simulink model "amuntitled"  (R2016a)
settings: Solver=FixedStepDiscrete  SolverMode=SingleTasking  StartTime=0.0  StopTime=4e-6  RelTol=1e-3
InitFcn:
  | %% DSPBuilder Start
  | alt_dspbuilder_update_model(bdroot)
  | %% DSPBuilder End
StartFcn:
  | %% DSPBuilder Start
  | alt_dspbuilder_hdlimport_prepare_for_simulation(bdroot)
  | %% DSPBuilder End
libraries: allblocks_alteradspbuilder2 x13
settings Model: Creator=ASUS  LastModifiedBy=ASUS

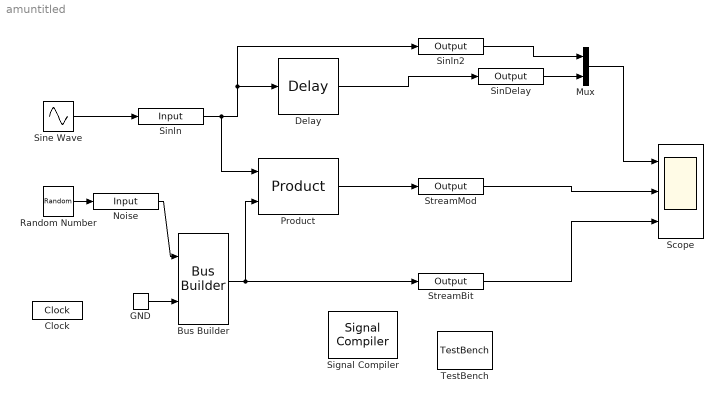
== system amuntitled ==
  Bus Builder : allblocks_alteradspbuilder2/Bus Builder  BusType=Signed Integer  bwl=2  bwr=1  pipeline_display=0
  Clock : allblocks_alteradspbuilder2/Clock  ClockPeriod=20  ClockPeriodUnit=ns  SampleTime=2.5e-008  ResetLatency=0  ResetRegisterCascadeDepth=0  SimulationStartCycle=5  PhaseOffset=0  Reset=aclr  ResetType=Active High  Export=off
  Delay : allblocks_alteradspbuilder2/Delay  pipeline=01  pipeline_display=1  ClockPhase=1  use_ena=off  use_sclr=off  allowFloatingPointOverride=on  logOutputs=off  logFile=D:\intelFPGA\18.0\quartus\dsp_builder\bin64\tb_amuntitled\amuntitled_Delay.fixedpointlog  use_init=off  reset_value=1
  GND : allblocks_alteradspbuilder2/GND  SpecifyClock=off
  Mux : Mux  Inputs=2
  Noise : allblocks_alteradspbuilder2/Input  iofile=D:\git\上传项目\tb_amuntitled\amuntitled_Noise.salt  BusType=Single Bit  bwl=8  bwr=0  SpecifyClock=off  PORTTYPE=Input  externalType=Inferred  allowFloatingPointOverride=on  logOutputs=off
  Product : allblocks_alteradspbuilder2/Product  BusType=Inferred  bwl=8  bwr=0  pipeline=0  pipeline_display=0  phase_selection=1  use_ena=off  use_aclr=off  UseLPM=off  UseDedicatedCircuitry=on  allowFloatingPointOverride=on  logOutputs=off  logFile=D:\intelFPGA\18.0\quartus\dsp_builder\bin64\tb_amuntitled\amuntitled_Product.fixedpointlog
  Random Number : RandomNumber  SampleTime=25e-9
  Scope : Scope  NumInputPorts=3
  Signal Compiler : allblocks_alteradspbuilder2/Signal Compiler  DeviceFamily=Cyclone IV GX  DeviceName=AUTO  DisableEarlyHDLGeneration=off  EnableSignalTap=off  SignalTapDepth=128  UseBoardBlock=off  StpUseDefaultClock=on  StpClock=Clock  ExportDir=D:\intelFPGA\18.0\quartus\dsp_builder  MAX10_ProgrammingMode=Internal Flash (SDM) Single Boot
  SinDelay : allblocks_alteradspbuilder2/Output  iofile=D:\git\上传项目\tb_amuntitled\amuntitled_SinDelay.capture  BusType=Signed Integer  bwl=16  bwr=0  externalType=Inferred  PORTTYPE=Output  allowFloatingPointOverride=on  logOutputs=off
  Sine Wave : Sin  SineType=Sample based  Amplitude=2^15-1  Samples=80  SampleTime=25e-9
  Sinln : allblocks_alteradspbuilder2/Input  iofile=D:\git\上传项目\tb_amuntitled\amuntitled_Sinln.salt  BusType=Signed Integer  bwl=16  bwr=0  SpecifyClock=off  PORTTYPE=Input  externalType=Inferred  allowFloatingPointOverride=on  logOutputs=off
  Sinln2 : allblocks_alteradspbuilder2/Output  iofile=D:\git\上传项目\tb_amuntitled\amuntitled_Sinln2.capture  BusType=Signed Integer  bwl=16  bwr=0  externalType=Inferred  PORTTYPE=Output  allowFloatingPointOverride=on  logOutputs=off
  StreamBit : allblocks_alteradspbuilder2/Output  iofile=D:\git\上传项目\tb_amuntitled\amuntitled_StreamBit.capture  BusType=Single Bit  bwl=19  bwr=0  externalType=Inferred  PORTTYPE=Output  allowFloatingPointOverride=on  logOutputs=off
  StreamMod : allblocks_alteradspbuilder2/Output  iofile=D:\git\上传项目\tb_amuntitled\amuntitled_StreamMod.capture  BusType=Signed Integer  bwl=19  bwr=0  externalType=Inferred  PORTTYPE=Output  allowFloatingPointOverride=on  logOutputs=off
  TestBench : allblocks_alteradspbuilder2/TestBench  enable=on  advancedMode=on  modelSimGui=on  genNCSimScripts=off  maxDisplayErrors=10  mismatchErrorLevel=Error  simdatafile=D:\intelFPGA\18.0\quartus\dsp_builder\bin64\tb_amuntitled\amuntitled.simdata.tcl
  wires:
  Sine Wave/1 -> Sinln/1
  Sinln/1 -> Product/1, Sinln2/1, Delay/1
  Delay/1 -> SinDelay/1
  Sinln2/1 -> Mux/1
  SinDelay/1 -> Mux/2
  Bus Builder/1 -> Product/2, StreamBit/1
  GND/1 -> Bus Builder/2
  Random Number/1 -> Noise/1
  Noise/1 -> Bus Builder/1
  Product/1 -> StreamMod/1
  Mux/1 -> Scope/1
  StreamMod/1 -> Scope/2
  StreamBit/1 -> Scope/3
